simulink model "MBD_Subsystem_Mask"  (R2021b)
settings: Solver=FixedStepDiscrete  StartTime=0.0  StopTime=10.0  FixedStep=0.001  RelTol=1e-3
settings Model: Creator=waleed.elshemy  LastModifiedBy=waleed.elshemy
settings OptimizationCC: DefaultParameterBehavior=Inlined  UseDivisionForNetSlopeComputation=on  GainParamInheritBuiltInType=on  UseFloatMulNetSlope=on  InlineInvariantSignals=on  PassReuseOutputArgsAs=Individual arguments  ZeroExternalMemoryAtStartup=off  ZeroInternalMemoryAtStartup=off  NoFixptDivByZeroProtection=on  EfficientFloat2IntCast=on  LifeSpan=1  OptimizeBlockOrder=speed  DifferentSizesBufferReuse=on  EfficientTunableParamExpr=on
settings DebuggingCC: ParameterTunabilityLossMsg=error
settings HardwareCC: ProdLongLongMode=on
settings SFSimCC: MATLABDynamicMemAlloc=off
settings RTWCC: Description=Embedded Coder  SystemTargetFile=ert.tlc  TemplateMakefile=ert_default_tmf
settings CodeAppCC: ForceParamTrailComments=on  IgnoreCustomStorageClasses=off  OperatorAnnotations=on  SimulinkDataObjDesc=on  SFDataObjDesc=on  CustomSymbolStrGlobalVar=rt$N$M  CustomSymbolStrType=$N$M  CustomSymbolStrFcn=$N$M$F  CustomSymbolStrMacro=$N$M  InsertBlockDesc=on
settings ERTTargetCC: TargetLangStandard=C99 (ISO)  GenerateSampleERTMain=on  IncludeMdlTerminateFcn=off  CombineSignalStateStructs=on  SupportComplex=off  SupportContinuousTime=on  InlinedParameterPlacement=NonHierarchical  ERTCustomFileTemplate=example_file_process.tlc

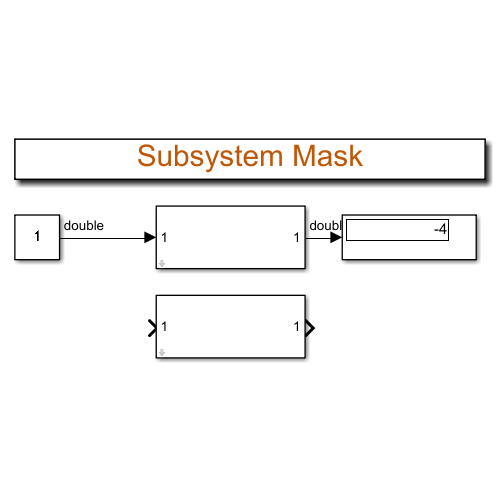
[thumbnail: Simulink's stored preview of the top-level diagram]
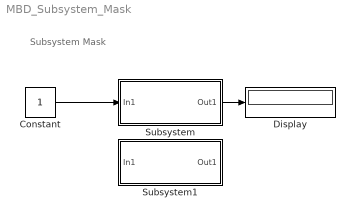
== system MBD_Subsystem_Mask ==
  note: Subsystem Mask
  Constant : Constant
  Display : Display
  Subsystem : Subsystem  mask{Shifting_Value=5, Scaling_Value=0, Min_Value=[], Max_Value=[], Parameter5=1}
      mask prompts: Shifting_Value "Shifting Value"; Min_Value "Min"; Max_Value "Max"; Parameter5 "Combo Box Options"
      mask TypeOptions Parameter5: 1 | 2 | 3 | 4 | 5
      mask DialogControl DescTextVar Prompt: This mask shifts and scales the input>
      mask DialogControl Container7 Prompt: Main
      mask DialogControl Control2 Prompt: Scaling Value
      mask DialogControl Container8 Prompt: Signal
  Subsystem1 : Subsystem  mask{Shifting_Value=6, Scaling_Value=4.200, Min_Value=[], Max_Value=[], Parameter5=1}
      mask prompts: Shifting_Value "Shifting Value"; Min_Value "Min"; Max_Value "Max"; Parameter5 "Combo Box Options"
      mask TypeOptions Parameter5: 1 | 2 | 3 | 4 | 5
      mask DialogControl DescTextVar Prompt: This mask shifts and scales the input>
      mask DialogControl Container7 Prompt: Main
      mask DialogControl Control2 Prompt: Scaling Value
      mask DialogControl Container8 Prompt: Signal
  wires:
  Constant/1 -> Subsystem/1(In1)
  Subsystem/1(Out1) -> Display/1

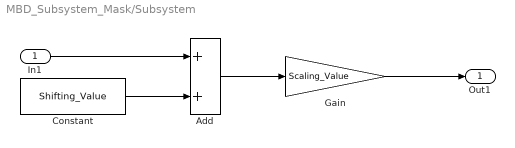
== system MBD_Subsystem_Mask/Subsystem ==
  In1 : Inport
  Add : Sum
  Constant : Constant  Value=Shifting_Value
  Gain : Gain  Gain=Scaling_Value
  Out1 : Outport
  wires:
  In1/1 -> Add/1
  Constant/1 -> Add/2
  Add/1 -> Gain/1
  Gain/1 -> Out1/1

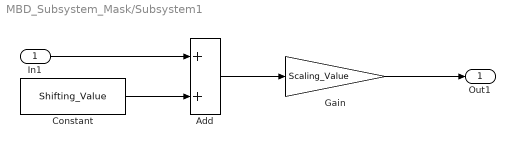
== system MBD_Subsystem_Mask/Subsystem1 ==
  In1 : Inport
  Add : Sum
  Constant : Constant  Value=Shifting_Value
  Gain : Gain  Gain=Scaling_Value
  Out1 : Outport
  wires:
  In1/1 -> Add/1
  Constant/1 -> Add/2
  Add/1 -> Gain/1
  Gain/1 -> Out1/1
